simulink model "Lab5Pt2"  (R2020b)
settings: Solver=VariableStepDiscrete  StartTime=0.0  StopTime=3.1  MaxStep=0.001  RelTol=1e-3
undefined symbols (not defined in the file or in its folder): f
libraries: dspfdesign x1
settings Model: Creator=abenkum  LastModifiedBy=abenkum

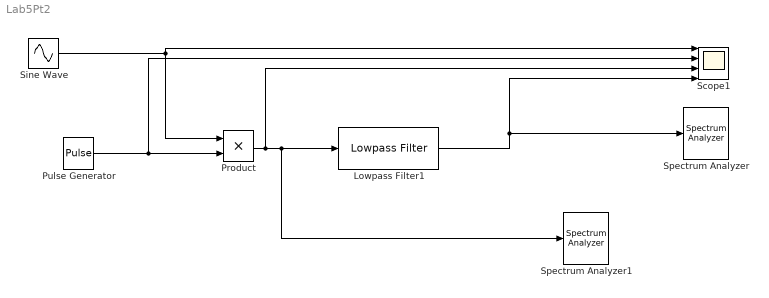
== system Lab5Pt2 ==
  Lowpass Filter1 : dspfdesign/Lowpass Filter  FilterType=IIR  DesignForMinimumOrder=on  FilterOrder=50  PassbandFrequency=4.9  StopbandFrequency=5.1  PassbandRipple=0.1  StopbandAttenuation=80  InheritSampleRate=off  SampleRate=1000  SimulateUsing=Interpreted execution  roundingMode=Floor  coeffsDataTypeStr=fixdt(1,16)
  Product : Product
  Pulse Generator : DiscretePulseGenerator  Period=100  SampleTime=0.001
  Scope1 : Scope  NumInputPorts=4
  Sine Wave : Sin  SineType=Sample based  Frequency=2*pi*f  Phase=pi/2  Samples=125  SampleTime=0.001
  Spectrum Analyzer : SpectrumAnalyzer
  Spectrum Analyzer1 : SpectrumAnalyzer
  wires:
  Pulse Generator/1 -> Scope1/2, Product/2
  Product/1 -> Scope1/3, Spectrum Analyzer1/1, Lowpass Filter1/1
  Sine Wave/1 -> Scope1/1, Product/1
  Lowpass Filter1/1 -> Scope1/4, Spectrum Analyzer/1
